simulink model "MPC_regul"  (R2017a)
settings: Solver=VariableStepAuto  StartTime=0.0  StopTime=10.0  RelTol=1e-3
settings Model: Creator=sverreknutsen  LastModifiedBy=sverreknutsen

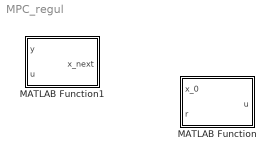
== system MPC_regul ==
  MATLAB Function : MATLAB Function  TreatAsAtomicUnit=on
  MATLAB Function1 : MATLAB Function  TreatAsAtomicUnit=on

== matlab function MPC_regul/MATLAB Function1 ==
  data: y input; u input; x_next output
function x_next = kalmanFilter(y,u)
persistent x;
persistent P;
persistent K;
persistent R;

if(isempty(x))
    x=0;
else
A=linearA(x);
yhat=C*x;
R=Qe+C*P*C';
K=(A*P*C')/(Qe+C*P*C')
x=A*x+B*u+K*(y-yhat);
P=A*P*A'+Qv-K*R*K';
end

== matlab function MPC_regul/MATLAB Function ==
  data: x_0 input; u output; r input
function u = MPC(x_0,r)

x10=0;
x20=0;
x30=pi/4;
x40=0;
x50=u10/k1;
x60=u20/k2;
u10=10;
u20=10;
[A,B]=linearization(x10,x20,x30,x40,x50,x60,u10,u20);

%setup opt problem
params.A=A;
params.B=B;
params.Q=eye(6);
params.R=eye(2);
params.u_max=10;
params.u_min=-10;
params.x_0=[x10,x20,x30,x40,x50,x60]';

% Create a new settings structure, with some example settings.
settings.verbose = 0;  % disable output of solver progress.
settings.max_iters = 10;  % reduce the maximum iteration count, from 25.
settings.eps = 0.1;  % reduce the required objective tolerance, from 1e-6.
settings.resid_tol = 1e-2;  % reduce the required residual tolerances, from 1e-4.

% solv
[vars, status] = csolve(params, settings);
u=vars.u_1;
x=vars.x;
